simulink model "inverted_double_pendulum_on_a_cart_model"  (R2019b)
settings: Solver=ode15s  StartTime=0.0  StopTime=0.5  FixedStep=0.05  RelTol=0.4
values from neighbouring files (symbols this model uses):
  g = 9.8    [inverted_double_pendulum_on_a_cart.m]    (also in inverted_double_pendulum_on_a_cart_params.m = 9.81)
  l1 = 20    [inverted_double_pendulum_on_a_cart.m]    (also in inverted_double_pendulum_on_a_cart_params.m)
  l2 = 10    [inverted_double_pendulum_on_a_cart.m]    (also in inverted_double_pendulum_on_a_cart_params.m)
  m0 = 1000    [inverted_double_pendulum_on_a_cart.m]    (also in inverted_double_pendulum_on_a_cart_params.m)
  m1 = 100    [inverted_double_pendulum_on_a_cart.m]    (also in inverted_double_pendulum_on_a_cart_params.m)
  m2 = 100    [inverted_double_pendulum_on_a_cart.m]    (also in inverted_double_pendulum_on_a_cart_params.m)
settings Model: Creator=Jerrar  LastModifiedBy=Eugene
settings DataIOCC: ReturnWorkspaceOutputs=off
settings DebuggingCC: ArithmeticOperatorsInVariantConditions=warning
settings SFSimCC: SimUseLocalCustomCode=off  CustomCodeUndefinedFunction=UseInterfaceOnly
settings RTWCC: RTWUseLocalCustomCode=off

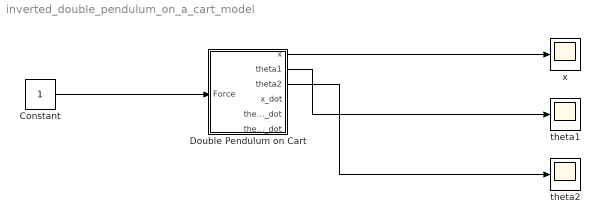
== system inverted_double_pendulum_on_a_cart_model ==
  Constant : Constant
  Double Pendulum on Cart : Subsystem
  theta1 : Scope
  theta2 : Scope
  x : Scope
  wires:
  Double Pendulum on Cart/1(x) -> x/1
  Double Pendulum on Cart/2(theta1) -> theta1/1
  Double Pendulum on Cart/3(theta2) -> theta2/1
  Constant/1 -> Double Pendulum on Cart/1(Force)

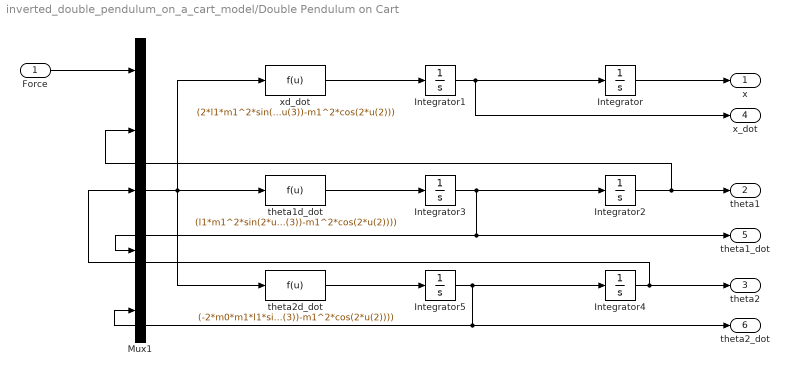
== system inverted_double_pendulum_on_a_cart_model/Double Pendulum on Cart ==
  Force : Inport
  Integrator{,1..5} (6 alike) : Integrator
  Mux1 : Mux  Inputs=5
  theta1d_dot : Fcn  Expr=(l1*m1^2*sin(2*u(2))+l1*m1*m2*sin(2*u(2))+l2*m0*m2*l2*sin(2*u(2)-2*u(3)))*u(4)^2-(m1*m2*l2*sin(u(2)+u(3))+m1*m2*l2*sin(u(2)-u(3))+2*m0*m2*l2*sin(u(2)-u(3)))*u(5)^2-m0*m1*(-2*sin(u(2))-m0*m2*sin(u(2))-2*m1^2*sin(u(2))-2*m1*m2*sin(u(2))-m0*m2*sin(u(2))-2*u(3))*g+(2*m0*m1*cos(u(2))+m0*m2*cos(u(2))-m0*m2*cos(u(2)-u(3)))*u(1)/(l1*(m1^2+2*m0*m1+m0*m2+m1*m2-m0*m2*cos(2*u(2)-2*u(3))-m1^2*cos(2*u(2))))
  theta2d_dot : Fcn  Expr=(-2*m0*m1*l1*sin(u(2)-u(3))-2*m0*m2*l2*sin(u(2)-u(3)))*u(4)^2+m0*m2*l2*sin(2*u(2)-2*u(3))*u(5)^2-(m0*m1*sin(2*u(2)-u(3))-m0*m1*sin(u(3))+m0*m2*sin(2*u(2)-u(3))-m0*m2*sin(u(3)))*g+(m0*m1*cos(u(3))-m0*m1*cos(2*u(2)-u(3))+m0*m2*cos(u(3))-m0*m2*cos(2*u(2)-u(3)))*u(1)/(l2*(m1^2+2*m0*m1+m0*m2+m1*m2-m0*m2*cos(2*u(2)-2*u(3))-m1^2*cos(2*u(2))))
  xd_dot : Fcn  Expr=(2*l1*m1^2*sin(u(2))+2*l1*m1*m2*sin(u(2)))*u(4)^2-(m1*m2*l2*sin(2*u(2)-u(3))+m1*m2*l2*sin(u(3)))*u(5)^2-(-m1^2*sin(2*u(2))-m1*m2*sin(2*u(2)))*g+(2*m0*m1+m0*m2-m0*m2*cos(2*u(2)-2*u(3)))*u(1)/(m1^2+2*m0*m1+m0*m2+m1*m2-m0*m2*cos(2*u(2)-2*u(3))-m1^2*cos(2*u(2)))
  x : Outport  VectorParamsAs1DForOutWhenUnconnected=off
  theta1 : Outport  Port=2  VectorParamsAs1DForOutWhenUnconnected=off
  theta2 : Outport  Port=3  VectorParamsAs1DForOutWhenUnconnected=off
  x_dot : Outport  Port=4  VectorParamsAs1DForOutWhenUnconnected=off
  theta1_dot : Outport  Port=5  VectorParamsAs1DForOutWhenUnconnected=off
  theta2_dot : Outport  Port=6  VectorParamsAs1DForOutWhenUnconnected=off
  wires:
  Integrator4/1 -> theta2/1, Mux1/3
  Integrator/1 -> x/1
  Integrator3/1 -> theta1_dot/1, Mux1/4, Integrator2/1
  Integrator5/1 -> Mux1/5, theta2_dot/1, Integrator4/1
  theta2d_dot/1 -> Integrator5/1
  Integrator1/1 -> Integrator/1, x_dot/1
  Force/1 -> Mux1/1
  xd_dot/1 -> Integrator1/1
  Integrator2/1 -> Mux1/2, theta1/1
  theta1d_dot/1 -> Integrator3/1
  Mux1/1 -> theta2d_dot/1, xd_dot/1, theta1d_dot/1
